simulink model "tts2"  (R2015a)
settings: Solver=ode45  StartTime=0.0  StopTime=7000.0  RelTol=1e-3
values from neighbouring files (symbols this model uses):
  alpha_constant = 0.5    [tts_model.m]
  beta = 0.37    [averagedRelayOutput.m]    (also in bursting_linearised.m = 0.27; compareApproximations.m = 1.5; fastSlow.m; fast_nullcline_winged_cusp.m = 0.5)
  delta = 0.5    [averagedRelayOutput.m]    (also in bursting_linearised.m; compareApproximations.m; fastSlow.m; fast_nullcline_winged_cusp.m)
  fast_plant_X0 = -1.0    (= -1)    [averagedRelayOutput.m]    (also in bursting_linearised.m = -1.05; fastSlow.m; fast_nullcline_winged_cusp.m; hRose.m = 0)
  gamma = 0    [averagedRelayOutput.m]    (also in bursting_linearised.m = 1; compareApproximations.m = 1; fastSlow.m; fast_nullcline_winged_cusp.m = 1)
  slow_plant_X0 = -1.0    (= -1)    [averagedRelayOutput.m]    (also in bursting_linearised.m = -1.05; fastSlow.m; fast_nullcline_winged_cusp.m = -2; hRose.m = -10)
  ts = 1    [averagedRelayOutput.m]    (also in bursting_linearised.m; compareApproximations.m; fastSlow.m; fast_nullcline_winged_cusp.m)
  tus = 800    [averagedRelayOutput.m]    (also in bursting_linearised.m = 200; fastSlow.m; manParamsNullclines.m; manipulateParameters.m = getappdata(hObject.Parent,'tus'))
  ultra_slow_plant_X0 = 0.45    [averagedRelayOutput.m]    (also in bursting_linearised.m = 0; fastSlow.m; hRose.m = 2000; manParamsNullclines.m)
settings Model: CovModelRefEnable=off  Creator=rajiv  LastModifiedBy=ra428
settings DataIOCC: SaveFormat=Dataset
settings HardwareCC: ProdBitPerPointer=64  ProdLargestAtomicFloat=Float  ProdIntDivRoundTo=Zero  ProdEndianess=LittleEndian  ProdHWDeviceType=Specified
settings GRTTargetCC: GeneratePreprocessorConditionals=Use local settings

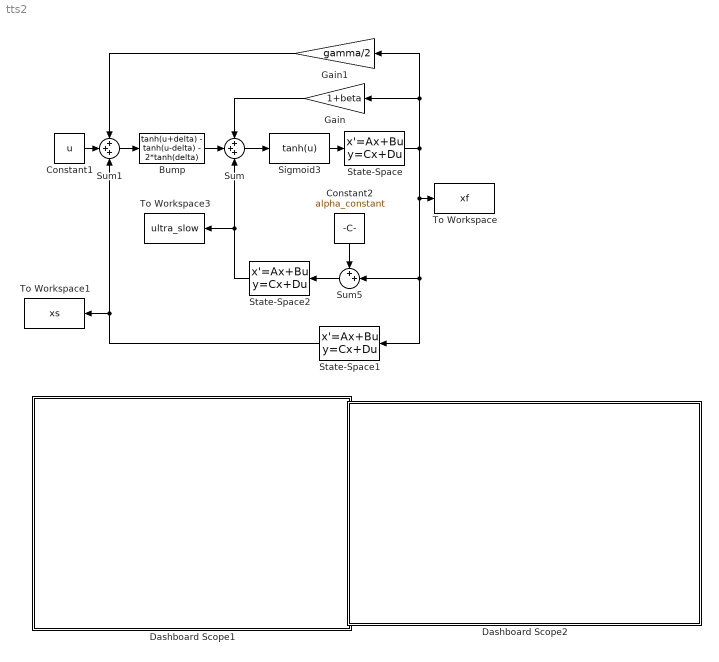
== system tts2 ==
  Bump : Fcn  Expr="tanh(u+delta) -  tanh(u-delta) - 2*tanh(delta)"
  Constant1 : Constant  Value=u
  Constant2 : Constant  Value=alpha_constant
  Dashboard Scope1 : Subsystem  DialogController=hmiCreateDDGDialog  IsWebBlock=on  mask(MathWorksWebBlock){webBlockId=4fc1403d-1d7a-4d36-bf15-73389c411ac4, webBlockType=sdiscope, ShowInitialText=on, HMISrcModelName=tts2}
      mask prompts: webBlockId "WebBlock Id"; webBlockType "WebBlock Type"; HMISrcModelName "Source Model"
      mask Help: helpview([docroot '/mapfiles/simulink.map'], 'hmi_scope')
      mask Display:
      | if strcmp(get_param(bdroot(gcb),'BlockDiagramType'), 'library')
      |     image([(matlabroot) '/toolbox/simulink/hmi/icons/DashboardScope.png']);
      | end
  Dashboard Scope2 : Subsystem  DialogController=hmiCreateDDGDialog  IsWebBlock=on  mask(MathWorksWebBlock){webBlockId=6bca0d0a-91f5-4129-a667-56d3cf01a8ea, webBlockType=sdiscope, ShowInitialText=on, HMISrcModelName=tts2}
      mask prompts: webBlockId "WebBlock Id"; webBlockType "WebBlock Type"; HMISrcModelName "Source Model"
      mask Help: helpview([docroot '/mapfiles/simulink.map'], 'hmi_scope')
      mask Display:
      | if strcmp(get_param(bdroot(gcb),'BlockDiagramType'), 'library')
      |     image([(matlabroot) '/toolbox/simulink/hmi/icons/DashboardScope.png']);
      | end
  Gain : Gain  Gain=1+beta
  Gain1 : Gain  Gain=gamma/2
  Sigmoid3 : Fcn  Expr=tanh(u)
  State-Space : StateSpace  A=-1/tf  B=1/tf  D=0  X0=fast_plant_X0
  State-Space1 : StateSpace  A=-1/ts  B=1/ts  D=0  X0=slow_plant_X0
  State-Space2 : StateSpace  A=-1/tus  B=-1/tus  D=0  X0=ultra_slow_plant_X0
  Sum : Sum  Inputs=+++
  Sum1 : Sum  Inputs=+++
  Sum5 : Sum  Inputs=++|
  To Workspace : ToWorkspace  VariableName=xf  SaveFormat=Timeseries  SampleTime=-1
  To Workspace1 : ToWorkspace  VariableName=xs  SaveFormat=Timeseries  SampleTime=-1
  To Workspace3 : ToWorkspace  VariableName=ultra_slow  SaveFormat=Timeseries  SampleTime=-1
  wires:
  Sum/1 -> Sigmoid3/1
  Gain/1 -> Sum/1
  State-Space1/1 -> Sum1/3, To Workspace1/1
  Gain1/1 -> Sum1/1
  Sigmoid3/1 -> State-Space/1
  State-Space/1 -> Gain/1, Gain1/1, To Workspace/1, State-Space1/1, Sum5/2
  Constant1/1 -> Sum1/2
  Sum1/1 -> Bump/1
  Bump/1 -> Sum/2
  State-Space2/1 -> Sum/3, To Workspace3/1
  Sum5/1 -> State-Space2/1
  Constant2/1 -> Sum5/1

== system tts2/Dashboard Scope1 ==

== system tts2/Dashboard Scope2 ==
